simulink model "Simulink_Model_Plate"  (R2021a)
settings: Solver=VariableStepAuto  StartTime=0.0  StopTime=500  RelTol=1e-3
libraries: simulink x5
settings Model: Creator=Alfonso  LastModifiedBy=Alfonso
settings SolverCC: AlgebraicLoopSolver=TrustRegion
settings DataIOCC: ReturnWorkspaceOutputs=off
settings DebuggingCC: SFMachineParentedDataDiag=warning  ArithmeticOperatorsInVariantConditions=warning
settings SFSimCC: SimUseLocalCustomCode=off  CustomCodeUndefinedFunction=UseInterfaceOnly
settings RTWCC: RTWUseLocalCustomCode=off

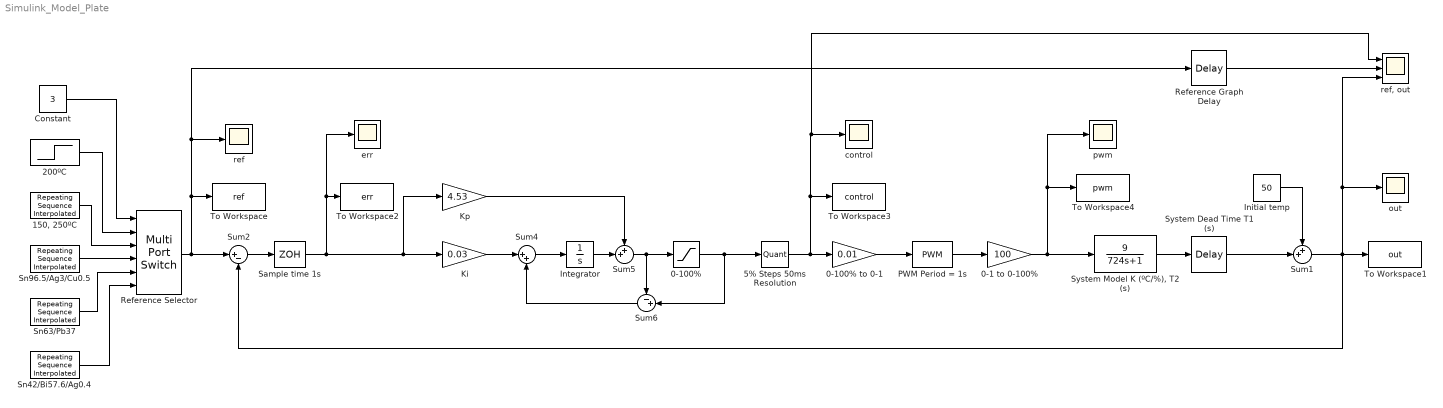
== system Simulink_Model_Plate ==
  0-1 to 0-100% : Gain  Gain=100
  0-100% : Saturate  UpperLimit=100  LowerLimit=0
  0-100% to 0-1 : Gain  Gain=0.01
  "150, 250ºC" : simulink/Sources/Repeating Sequence Interpolated  OutValues=[150 150 250 250].'  TimeValues=[0 500 501 1000].'  LookUpMeth=Interpolation-Use End Values  tsamp=0.01  OutMin=[]  OutMax=[]  OutDataTypeStr=double  OutputDataTypeScalingMode=double  OutDataType=fixdt(0,8)  OutScaling=2^-10
  200ºC : Step  Time=0  Before=50  After=200  SampleTime=0.01
  5% Steps 50ms Resolution : Quantizer  QuantizationInterval=5
  Constant : Constant  Value=3
  Initial temp : Constant  Value=50
  Integrator : Integrator
  Ki : Gain  Gain=0.03
  Kp : Gain  Gain=4.53
  PWM Period = 1s : simulink/Discontinuities/PWM  DisableCoverage=on  Period=1  DisallowZeroDutyCycle=off  RunAtFixedTimeIntervals=off  SampleTime=0.1
  Reference Selector : MultiPortSwitch  Inputs=5
  Reference Graph Delay : TransportDelay  DelayTime=0
  Sample time 1s : ZeroOrderHold
  Sn42/Bi57.6/Ag0.4 : simulink/Sources/Repeating Sequence Interpolated  OutValues=[50 100 130 170 170 50 50].'  TimeValues=[0 50 140 190 220 280 500].'  LookUpMeth=Interpolation-Use End Values  tsamp=0.01  OutMin=[]  OutMax=[]  OutDataTypeStr=double  OutputDataTypeScalingMode=double  OutDataType=fixdt(0,8)  OutScaling=2^-10
  Sn63/Pb37 : simulink/Sources/Repeating Sequence Interpolated  OutValues=[50 120 150 220 220 50 50].'  TimeValues=[0 70 160 250 280 360 500].'  LookUpMeth=Interpolation-Use End Values  tsamp=0.01  OutMin=[]  OutMax=[]  OutDataTypeStr=double  OutputDataTypeScalingMode=double  OutDataType=fixdt(0,8)  OutScaling=2^-10
  Sn96.5/Ag3/Cu0.5 : simulink/Sources/Repeating Sequence Interpolated  OutValues=[50 150 180 250 250 50 50].'  TimeValues=[0 80 140 230 270 370 500].'  LookUpMeth=Interpolation-Use End Values  tsamp=0.01  OutMin=[]  OutMax=[]  OutDataTypeStr=double  OutputDataTypeScalingMode=double  OutDataType=fixdt(0,8)  OutScaling=2^-10
  Sum1 : Sum  Inputs=++|
  Sum2 : Sum  Inputs=|+-
  Sum4 : Sum  Inputs=|++
  Sum5 : Sum  Inputs=++|
  Sum6 : Sum  Inputs=-+|
  System Dead Time T1 (s) : TransportDelay  DelayTime=16
  "System Model K (ºC/%), T2 (s)" : TransferFcn  Numerator=[9]  Denominator=[724 1]
  To Workspace : ToWorkspace  VariableName=ref  SaveFormat=Timeseries  SampleTime=-1
  To Workspace1 : ToWorkspace  VariableName=out  SaveFormat=Timeseries  SampleTime=-1
  To Workspace2 : ToWorkspace  VariableName=err  SaveFormat=Timeseries  SampleTime=-1
  To Workspace3 : ToWorkspace  VariableName=control  SaveFormat=Timeseries  SampleTime=-1
  To Workspace4 : ToWorkspace  VariableName=pwm  SaveFormat=Timeseries  SampleTime=-1
  "control " : Scope
  err : Scope
  out : Scope
  pwm : Scope
  ref : Scope
  "ref, out" : Scope  NumInputPorts=3
  wires:
  Ki/1 -> Sum4/1
  Kp/1 -> Sum5/1
  Sum6/1 -> Sum4/2
  Integrator/1 -> Sum5/2
  Sum4/1 -> Integrator/1
  Sum5/1 -> 0-100%/1, Sum6/1
  0-1 to 0-100%/1 -> "System Model K (ºC/%), T2 (s)"/1, pwm/1, To Workspace4/1
  0-100% to 0-1/1 -> PWM Period = 1s/1
  PWM Period = 1s/1 -> 0-1 to 0-100%/1
  "System Model K (ºC/%), T2 (s)"/1 -> System Dead Time T1 (s)/1
  Constant/1 -> Reference Selector/1
  200ºC/1 -> Reference Selector/2
  "150, 250ºC"/1 -> Reference Selector/3
  Sn96.5/Ag3/Cu0.5/1 -> Reference Selector/4
  Sn63/Pb37/1 -> Reference Selector/5
  Sn42/Bi57.6/Ag0.4/1 -> Reference Selector/6
  System Dead Time T1 (s)/1 -> Sum1/2
  Initial temp/1 -> Sum1/1
  Sum1/1 -> "ref, out"/3, out/1, To Workspace1/1, Sum2/2
  5% Steps 50ms Resolution/1 -> To Workspace3/1, "ref, out"/1, "control "/1, 0-100% to 0-1/1
  Sum2/1 -> Sample time 1s/1
  0-100%/1 -> Sum6/2, 5% Steps 50ms Resolution/1
  Sample time 1s/1 -> To Workspace2/1, err/1, Kp/1, Ki/1
  Reference Selector/1 -> Sum2/1, To Workspace/1, Reference Graph Delay/1, ref/1
  Reference Graph Delay/1 -> "ref, out"/2
